simulink model "AirCooledDataCenterTemperatureProfile"  (R2025b)
settings: Solver=daessc  StartTime=0.0  StopTime=24*3600  MaxStep=1  RelTol=1e-3  AbsTol=1e-3
PreLoadFcn:
  | if ~exist("airCooledDataCenter")
  |     setModelParam;
  | end
undefined symbols (not defined in the file or in its folder): airCooledDataCenter, DiscIntNeverNeededParam, value
libraries: fl_lib x166, nesl_utility x25, datacenter_lib x24, simulink_extras x9
(part 1 of 4)
settings Model: Creator=vikrants  LastModifiedBy=vikrants
settings SolverCC: AutoScaleAbsTol=off  MaxConsecutiveMinStep=3  AlgebraicLoopSolver=TrustRegion  MaxZcPerStep=1.0
settings DataIOCC: SaveOutput=off  DSMLogging=off  SaveTime=off  ReturnWorkspaceOutputs=off  SignalLoggingName=logsout_AirCooledDataCenterTprofile
settings DebuggingCC: UnconnectedInputMsg=warning  UnconnectedOutputMsg=warning  UnconnectedLineMsg=warning  SymbolicDimsDataTypeCodeGenerationDiagnostic=none
settings ModelReferenceCC: EnableRefExpFcnMdlSchedulingChecks=on
settings SFSimCC: CustomCodeUndefinedFunction=UseInterfaceOnly
settings RTWCC: GPUComputeCapability=3.5  DLArmComputeVersion=19.05
settings SimscapeCC: SimscapeLogSimulationStatistics=on  SimscapeLogDataHistory=10000.0

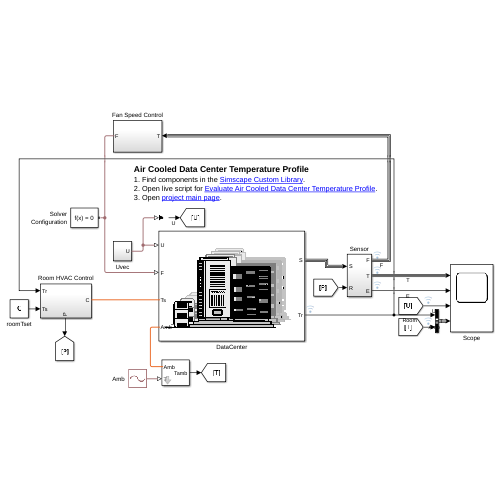
[thumbnail: Simulink's stored preview of the top-level diagram]
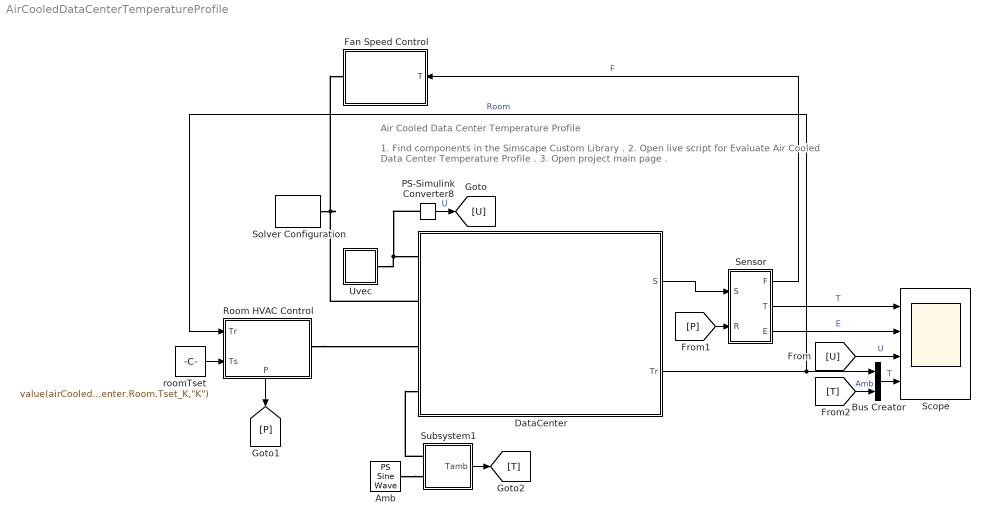
== system AirCooledDataCenterTemperatureProfile ==
  note: Air Cooled Data Center Temperature Profile
  note: 1. Find components in the Simscape Custom Library .
      | 2. Open live script for Evaluate Air Cooled Data Center Temperature Profile .
      | 3. Open project main page .
  Amb : fl_lib/Physical Signals/Sources/PS Sine Wave  amplitude=1 K  bias="value(airCooledDataCenter.HeatTransfer.AmbientT,\"K\") K"  frequency_spec=foundation.enum.frequencySpec.frequencySI  frequency_SI=1/3600 Hz  frequency_angular=1 rad/s  phase=0 rad
      settings: InternalSimscapePortConfiguration="{\"Bottom\":[],\"Left\":[],\"Right\":[{\"id\":\"O\",\"label\":\"\",\"type\":\"output\"}],\"Top\":[]}"
  Bus Creator : BusCreator  Inputs=2
  DataCenter : Subsystem
      mask Display: image('datacenterLibIcon.png');
  Fan Speed Control : Subsystem
      settings: PortSchema="{\"entries\":[{\"content\":{\"sides\":[{\"content\":{\"connectorIds\":[\"LConn1\"]},\"type\":\"ConnectorPlacement.EquallySpacedRectSide\",\"uuid\":\"25bb085d-e973-4ed5-b016-3236384605d7\"},{\"content\":{\"connectorIds\":[\"In1\"],\"side\":\"RIGHT\"},\"type\":\"ConnectorPlacement.EquallySpacedRectSide\",\"uuid\":\"9c70bb1c-0b86-445b-9231-deb3b11a43cd\"},{\"content\":{\"side\":\"TOP\"},\"type\":\"ConnectorPlacement.EquallySpacedRectSide\",\"uuid\":\"a44df08c-50be-4908-a6d5-8f6a23919272\"}]},\"type\":\"ConnectorPlacement.EquallySpacedConnector\",\"uuid\":\"adee43dd-4b72-4470-a633-4adaea9baf7d\"}],\"packageUris\":[\"http://schema.mathworks.com/mf0/Connector/R2020b\"],\"version\":\"1.0\"}"
  PS-Simulink Converter8 : nesl_utility/PS-Simulink Converter  PhysicalDomain=network_engine_domain  SubClassName=ps_output  LeftPortType=input  RightPortType=output  PseudoPeriodic=off  Frequencies=[]  VectorFormat=inherit  Unit=inherit  AffineConversion=off
  Room HVAC Control : Subsystem
      settings: PortSchema="{\"entries\":[{\"content\":{\"sides\":[{\"content\":{\"connectorIds\":[\"In1\",\"In2\"]},\"type\":\"ConnectorPlacement.EquallySpacedRectSide\",\"uuid\":\"3724864a-83d6-4228-951d-7164f41f00c6\"},{\"content\":{\"connectorIds\":[\"RConn1\"],\"side\":\"RIGHT\"},\"type\":\"ConnectorPlacement.EquallySpacedRectSide\",\"uuid\":\"0a482fb7-33c2-448f-90c4-95efee70f83f\"},{\"content\":{\"side\":\"TOP\"},\"type\":\"ConnectorPlacement.EquallySpacedRectSide\",\"uuid\":\"deb1033d-adc7-41d0-9927-16876749a2b1\"},{\"content\":{\"connectorIds\":[\"Out1\"],\"side\":\"BOTTOM\"},\"type\":\"ConnectorPlacement.EquallySpacedRectSide\",\"uuid\":\"12511515-206f-4008-b3c0-49360f108e7c\"}]},\"type\":\"ConnectorPlacement.EquallySpacedConnector\",\"uuid\":\"be3e27ef-0111-44f1-89d2-5affe53329b4\"}],\"packageUris\":[\"http://schema.mathworks.com/mf0/Connector/R2020b\"],\"version\":\"1.0\"}"
  Scope : Scope  NumInputPorts=4
      settings: ActiveDisplayYMinimum=-123.69235993685102  ActiveDisplayYMaximum=1124.8547066596502
  Sensor : Subsystem
  Solver Configuration : nesl_utility/Solver Configuration  PhysicalDomain=network_engine_domain  SubClassName=solver  LeftPortType=input  RightPortType=generic  Tones=[]  Harmonics=[]  SimulateNoise=off  Profile=off  UseLocalSampling=off  EnableSwitchedLinearOptims=on  FrequencyDomain=off  UseCCode=off  RelTol=0.001  AbsTol=1e-06  MinStep=1e-09  ToWorkspace=off  RevertToSquareIcSolve=off  NumHomotopyIterations=100  PhasorMode=off  PhasorModeNumHarmonics=1  ConsistencySolver=NEWTON_XTOL_AFTER_FTOL  IndexReductionMethod=DerivativeReplacement  DoDC=off  ResidualTolerance=1e-09  ConsistencyTolSource=GLOBAL  ConsistencyAbsTol=0.001  ConsistencyRelTol=0.001  ConsistencyTolFactor=0.001  UseLocalSolver=off  LocalSolverChoice=NE_BACKWARD_EULER_ADVANCER  ResolveIndetEquations=on  FunctionEvalNumThread=1  LocalSolverSampleTime=0.001  DoFixedCost=off  MaxNonlinIter=3  MaxModeIter=2  ComputeImpulses=off  ImpulseIterations=2  LinearAlgebra=auto  LinearAlgebraNumThread=0  EquationFormulation=NE_TIME_EF  DelaysMemoryBudget=1024  AutomaticFiltering=on  FilteringTimeConstant=0.001  PartitionStorageMethod=AS_NEEDED  PartitionMemoryBudget=1024  PartitionMethod=ROBUST  MultibodyUseLocalSolver=off  MultibodyLocalSolverChoice=ODE1  MultibodyLocalSolverSampleTime=0.001
  Subsystem1 : Subsystem  mask{thermalR=0.01}
      mask prompts: thermalR "Thermal resistance (K/W)"
  Uvec : Subsystem
  roomTset : Constant  Value="value(airCooledDataCenter.Room.Tset_K,\"K\")"
  wires:
  DataCenter/1(S) -> Sensor/1(S)
  Sensor/2(T) -> Scope/1  "T"
  Sensor/3(E) -> Scope/2  "E"
  Sensor/1(F) -> Fan Speed Control/1(T)  "F"
  PS-Simulink Converter8/1 -> [U]  "U"
  [U] -> Scope/3  "U"
  DataCenter/2(Tr) -> Bus Creator/1, Room HVAC Control/1(Tr)  "Room"
  Subsystem1/1(Tamb) -> [T]
  [T] -> Bus Creator/2  "Amb"
  Bus Creator/1 -> Scope/4  "T"
  roomTset/1 -> Room HVAC Control/2(Ts)
  Room HVAC Control/1(P) -> [P]
  [P] -> Sensor/2(R)
  connections:
  Uvec/RConn1 -- PS-Simulink Converter8/LConn1 -- DataCenter/LConn1
  DataCenter/LConn2 -- Fan Speed Control/LConn1 -- Solver Configuration/RConn1
  Subsystem1/LConn1 -- DataCenter/LConn4
  Amb/RConn1 -- Subsystem1/LConn2
  Room HVAC Control/RConn1 -- DataCenter/LConn3

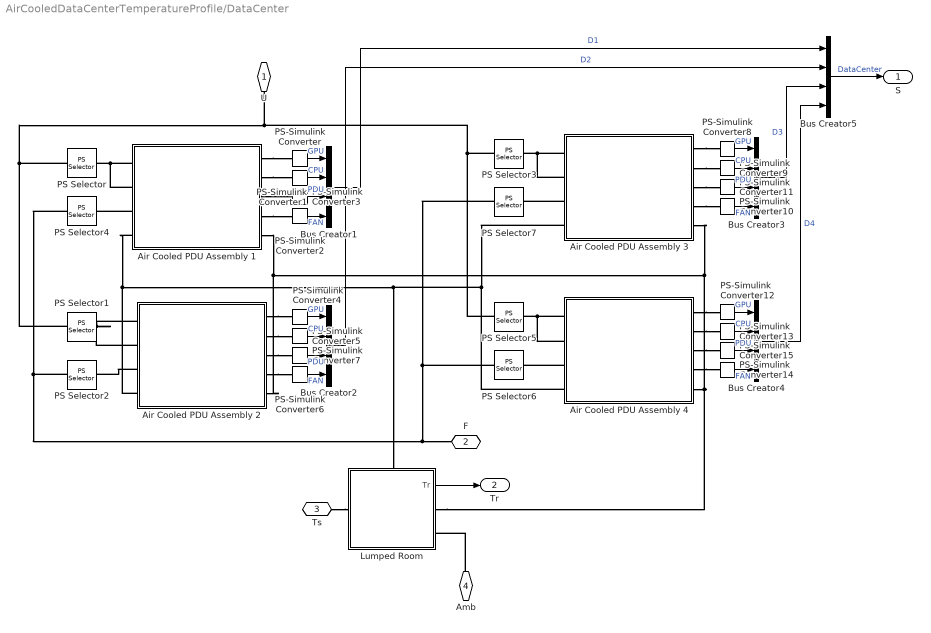
== system AirCooledDataCenterTemperatureProfile/DataCenter ==
  Air Cooled PDU Assembly 1 : Subsystem  mask{nAssembly=1, nRacks=4, nTrays=6, nFans=36, flowVec=[500:250:1500]*0.000472, prDropVec=[7000:250:8000], fanEffVec=[0.88, 0.89, 0.90, 0.895, 0.89], trayMass=8, trayCp=8000, trayThermalR=1e-3, nGPU=4, gpuTDPperDie=1200, gpuIdlePower=300, gpuHBMpower=80, gpuExponent=1.4, gpuHBMutil=0.7, gpuLeakage=1.5, gpuNominalDieT=350, gpuDieThermalC=50, gpuHeatSinkR=1e-3, gpuSurfArea=0.01, gpuAmbientR=1e-3, nCPU=2, cpuTDPperSocket=350, cpuIdlePower=80, cpuExponent=1.1, cpuLeakage=1.5, cpuNominalDieT=350, cpuDieThermalC=50, cpuHeatSinkR=1e-3, cpuSurfArea=0.01, cpuAmbientR=1e-3, initialT=value(airCooledDataCenter.HeatTransfer.InitialT,"K"), htc=value(airCooledDataCenter.HeatTransfer.HTC,"W/(K*m^2)")}
      mask prompts: nAssembly "Number of PDU + Fan assemblies (-)"; nRacks "Number of racks per PDU (-)"; nTrays "Number of IT trays per rack (-)"; nFans "Number of fans per assembly (-)"; flowVec "Fan flow rate vector (m^3/s)"; prDropVec "Fan pressure drop vector (Pa)"; fanEffVec "Fan efficiency vector, 0-1 (-)"; trayMass "Tray mass (kg)"; trayCp "Tray specific heat capacity (J/kg*K)"; trayThermalR "Tray to external thermal resistance (K/W)"; nGPU "Number of GPU per tray (-)"; gpuTDPperDie "GPU TDP per die (W)"; gpuIdlePower "GPU idle power (W)"; gpuHBMpower "HBM power per GPU (W)"; gpuExponent "GPU power utilization exponent (-)"; gpuHBMutil "HBM utilization as fraction of compute utilization (-)"; gpuLeakage "Leakage increase per K above nominal temperature (W/K)"; gpuNominalDieT "Nominal die temperature at TDP (K)"; gpuDieThermalC "GPU die thermal capacitance (J/K)"; gpuHeatSinkR "GPU die-heat-sink thermal resistance (K/W)"; gpuSurfArea "Surface area per die for ambient heat transfer (m^2)"; gpuAmbientR "GPU die-ambient thermal resistance (K/W)"; nCPU "Number of CPU per tray (-)"; cpuTDPperSocket "CPU TDP per socket (W)"; cpuIdlePower "CPU idle power per socket (W)"; cpuExponent "CPU power utilization exponent (-)"; cpuLeakage "Leakage increase per K above nominal temperature (W/K)"; cpuNominalDieT "Nominal die temperature at TDP (K)"; cpuDieThermalC "CPU die thermal capacitance (J/K)"; cpuHeatSinkR "CPU die-heat-sink thermal resistance (K/W)"; cpuSurfArea "Surface area per die for ambient heat transfer (m^2)"; cpuAmbientR "CPU die-ambient thermal resistance (K/W)"; initialT "Initial temperature (K)"; htc "Heat transfer coefficient to ambient (W/m^2.K)"
      settings: CopyFcn=set_param(gcbh,'LinkStatus','none');
      mask Help: web("DocumentationAirCooledPDUAssembly.html")
      mask DialogControl Container10 Prompt: PDU Racks
      mask DialogControl getRatingButton Prompt: Get Rating
      mask DialogControl Container11 Prompt: Fans
      mask DialogControl Container9 Prompt: IT Tray
      mask DialogControl Container6 Prompt: GPU
      mask DialogControl Container7 Prompt: CPU
      mask DialogControl Container8 Prompt: Initial Conditions
      mask Display: image('icon_AssemblyAirCooled.png');
  Air Cooled PDU Assembly 2 : Subsystem  mask{nAssembly=1, nRacks=4, nTrays=6, nFans=36, flowVec=[500:250:1500]*0.000472, prDropVec=[7000:250:8000], fanEffVec=[0.88, 0.89, 0.90, 0.895, 0.89], trayMass=8, trayCp=8000, trayThermalR=1e-3, nGPU=4, gpuTDPperDie=1200, gpuIdlePower=300, gpuHBMpower=80, gpuExponent=1.4, gpuHBMutil=0.7, gpuLeakage=1.5, gpuNominalDieT=350, gpuDieThermalC=50, gpuHeatSinkR=1e-3, gpuSurfArea=0.01, gpuAmbientR=1e-3, nCPU=2, cpuTDPperSocket=350, cpuIdlePower=80, cpuExponent=1.1, cpuLeakage=1.5, cpuNominalDieT=350, cpuDieThermalC=50, cpuHeatSinkR=1e-3, cpuSurfArea=0.01, cpuAmbientR=1e-3, initialT=value(airCooledDataCenter.HeatTransfer.InitialT,"K"), htc=value(airCooledDataCenter.HeatTransfer.HTC,"W/(K*m^2)")}
      mask prompts: nAssembly "Number of PDU + Fan assemblies (-)"; nRacks "Number of racks per PDU (-)"; nTrays "Number of IT trays per rack (-)"; nFans "Number of fans per assembly (-)"; flowVec "Fan flow rate vector (m^3/s)"; prDropVec "Fan pressure drop vector (Pa)"; fanEffVec "Fan efficiency vector, 0-1 (-)"; trayMass "Tray mass (kg)"; trayCp "Tray specific heat capacity (J/kg*K)"; trayThermalR "Tray to external thermal resistance (K/W)"; nGPU "Number of GPU per tray (-)"; gpuTDPperDie "GPU TDP per die (W)"; gpuIdlePower "GPU idle power (W)"; gpuHBMpower "HBM power per GPU (W)"; gpuExponent "GPU power utilization exponent (-)"; gpuHBMutil "HBM utilization as fraction of compute utilization (-)"; gpuLeakage "Leakage increase per K above nominal temperature (W/K)"; gpuNominalDieT "Nominal die temperature at TDP (K)"; gpuDieThermalC "GPU die thermal capacitance (J/K)"; gpuHeatSinkR "GPU die-heat-sink thermal resistance (K/W)"; gpuSurfArea "Surface area per die for ambient heat transfer (m^2)"; gpuAmbientR "GPU die-ambient thermal resistance (K/W)"; nCPU "Number of CPU per tray (-)"; cpuTDPperSocket "CPU TDP per socket (W)"; cpuIdlePower "CPU idle power per socket (W)"; cpuExponent "CPU power utilization exponent (-)"; cpuLeakage "Leakage increase per K above nominal temperature (W/K)"; cpuNominalDieT "Nominal die temperature at TDP (K)"; cpuDieThermalC "CPU die thermal capacitance (J/K)"; cpuHeatSinkR "CPU die-heat-sink thermal resistance (K/W)"; cpuSurfArea "Surface area per die for ambient heat transfer (m^2)"; cpuAmbientR "CPU die-ambient thermal resistance (K/W)"; initialT "Initial temperature (K)"; htc "Heat transfer coefficient to ambient (W/m^2.K)"
      settings: CopyFcn=set_param(gcbh,'LinkStatus','none');
      mask Help: web("DocumentationAirCooledPDUAssembly.html")
      mask DialogControl Container10 Prompt: PDU Racks
      mask DialogControl getRatingButton Prompt: Get Rating
      mask DialogControl Container11 Prompt: Fans
      mask DialogControl Container9 Prompt: IT Tray
      mask DialogControl Container6 Prompt: GPU
      mask DialogControl Container7 Prompt: CPU
      mask DialogControl Container8 Prompt: Initial Conditions
      mask Display: image('icon_AssemblyAirCooled.png');
  Air Cooled PDU Assembly 3 : Subsystem  mask{nAssembly=1, nRacks=4, nTrays=6, nFans=36, flowVec=[500:250:1500]*0.000472, prDropVec=[7000:250:8000], fanEffVec=[0.88, 0.89, 0.90, 0.895, 0.89], trayMass=8, trayCp=8000, trayThermalR=1e-3, nGPU=4, gpuTDPperDie=1200, gpuIdlePower=300, gpuHBMpower=80, gpuExponent=1.4, gpuHBMutil=0.7, gpuLeakage=1.5, gpuNominalDieT=350, gpuDieThermalC=50, gpuHeatSinkR=1e-3, gpuSurfArea=0.01, gpuAmbientR=1e-3, nCPU=2, cpuTDPperSocket=350, cpuIdlePower=80, cpuExponent=1.1, cpuLeakage=1.5, cpuNominalDieT=350, cpuDieThermalC=50, cpuHeatSinkR=1e-3, cpuSurfArea=0.01, cpuAmbientR=1e-3, initialT=value(airCooledDataCenter.HeatTransfer.InitialT,"K"), htc=value(airCooledDataCenter.HeatTransfer.HTC,"W/(K*m^2)")}
      mask prompts: nAssembly "Number of PDU + Fan assemblies (-)"; nRacks "Number of racks per PDU (-)"; nTrays "Number of IT trays per rack (-)"; nFans "Number of fans per assembly (-)"; flowVec "Fan flow rate vector (m^3/s)"; prDropVec "Fan pressure drop vector (Pa)"; fanEffVec "Fan efficiency vector, 0-1 (-)"; trayMass "Tray mass (kg)"; trayCp "Tray specific heat capacity (J/kg*K)"; trayThermalR "Tray to external thermal resistance (K/W)"; nGPU "Number of GPU per tray (-)"; gpuTDPperDie "GPU TDP per die (W)"; gpuIdlePower "GPU idle power (W)"; gpuHBMpower "HBM power per GPU (W)"; gpuExponent "GPU power utilization exponent (-)"; gpuHBMutil "HBM utilization as fraction of compute utilization (-)"; gpuLeakage "Leakage increase per K above nominal temperature (W/K)"; gpuNominalDieT "Nominal die temperature at TDP (K)"; gpuDieThermalC "GPU die thermal capacitance (J/K)"; gpuHeatSinkR "GPU die-heat-sink thermal resistance (K/W)"; gpuSurfArea "Surface area per die for ambient heat transfer (m^2)"; gpuAmbientR "GPU die-ambient thermal resistance (K/W)"; nCPU "Number of CPU per tray (-)"; cpuTDPperSocket "CPU TDP per socket (W)"; cpuIdlePower "CPU idle power per socket (W)"; cpuExponent "CPU power utilization exponent (-)"; cpuLeakage "Leakage increase per K above nominal temperature (W/K)"; cpuNominalDieT "Nominal die temperature at TDP (K)"; cpuDieThermalC "CPU die thermal capacitance (J/K)"; cpuHeatSinkR "CPU die-heat-sink thermal resistance (K/W)"; cpuSurfArea "Surface area per die for ambient heat transfer (m^2)"; cpuAmbientR "CPU die-ambient thermal resistance (K/W)"; initialT "Initial temperature (K)"; htc "Heat transfer coefficient to ambient (W/m^2.K)"
      settings: CopyFcn=set_param(gcbh,'LinkStatus','none');
      mask Help: web("DocumentationAirCooledPDUAssembly.html")
      mask DialogControl Container10 Prompt: PDU Racks
      mask DialogControl getRatingButton Prompt: Get Rating
      mask DialogControl Container11 Prompt: Fans
      mask DialogControl Container9 Prompt: IT Tray
      mask DialogControl Container6 Prompt: GPU
      mask DialogControl Container7 Prompt: CPU
      mask DialogControl Container8 Prompt: Initial Conditions
      mask Display: image('icon_AssemblyAirCooled.png');
  Air Cooled PDU Assembly 4 : Subsystem  mask{nAssembly=1, nRacks=4, nTrays=6, nFans=36, flowVec=[500:250:1500]*0.000472, prDropVec=[7000:250:8000], fanEffVec=[0.88, 0.89, 0.90, 0.895, 0.89], trayMass=8, trayCp=8000, trayThermalR=1e-3, nGPU=4, gpuTDPperDie=1200, gpuIdlePower=300, gpuHBMpower=80, gpuExponent=1.4, gpuHBMutil=0.7, gpuLeakage=1.5, gpuNominalDieT=350, gpuDieThermalC=50, gpuHeatSinkR=1e-3, gpuSurfArea=0.01, gpuAmbientR=1e-3, nCPU=2, cpuTDPperSocket=350, cpuIdlePower=80, cpuExponent=1.1, cpuLeakage=1.5, cpuNominalDieT=350, cpuDieThermalC=50, cpuHeatSinkR=1e-3, cpuSurfArea=0.01, cpuAmbientR=1e-3, initialT=value(airCooledDataCenter.HeatTransfer.InitialT,"K"), htc=value(airCooledDataCenter.HeatTransfer.HTC,"W/(K*m^2)")}
      mask prompts: nAssembly "Number of PDU + Fan assemblies (-)"; nRacks "Number of racks per PDU (-)"; nTrays "Number of IT trays per rack (-)"; nFans "Number of fans per assembly (-)"; flowVec "Fan flow rate vector (m^3/s)"; prDropVec "Fan pressure drop vector (Pa)"; fanEffVec "Fan efficiency vector, 0-1 (-)"; trayMass "Tray mass (kg)"; trayCp "Tray specific heat capacity (J/kg*K)"; trayThermalR "Tray to external thermal resistance (K/W)"; nGPU "Number of GPU per tray (-)"; gpuTDPperDie "GPU TDP per die (W)"; gpuIdlePower "GPU idle power (W)"; gpuHBMpower "HBM power per GPU (W)"; gpuExponent "GPU power utilization exponent (-)"; gpuHBMutil "HBM utilization as fraction of compute utilization (-)"; gpuLeakage "Leakage increase per K above nominal temperature (W/K)"; gpuNominalDieT "Nominal die temperature at TDP (K)"; gpuDieThermalC "GPU die thermal capacitance (J/K)"; gpuHeatSinkR "GPU die-heat-sink thermal resistance (K/W)"; gpuSurfArea "Surface area per die for ambient heat transfer (m^2)"; gpuAmbientR "GPU die-ambient thermal resistance (K/W)"; nCPU "Number of CPU per tray (-)"; cpuTDPperSocket "CPU TDP per socket (W)"; cpuIdlePower "CPU idle power per socket (W)"; cpuExponent "CPU power utilization exponent (-)"; cpuLeakage "Leakage increase per K above nominal temperature (W/K)"; cpuNominalDieT "Nominal die temperature at TDP (K)"; cpuDieThermalC "CPU die thermal capacitance (J/K)"; cpuHeatSinkR "CPU die-heat-sink thermal resistance (K/W)"; cpuSurfArea "Surface area per die for ambient heat transfer (m^2)"; cpuAmbientR "CPU die-ambient thermal resistance (K/W)"; initialT "Initial temperature (K)"; htc "Heat transfer coefficient to ambient (W/m^2.K)"
      settings: CopyFcn=set_param(gcbh,'LinkStatus','none');
      mask Help: web("DocumentationAirCooledPDUAssembly.html")
      mask DialogControl Container10 Prompt: PDU Racks
      mask DialogControl getRatingButton Prompt: Get Rating
      mask DialogControl Container11 Prompt: Fans
      mask DialogControl Container9 Prompt: IT Tray
      mask DialogControl Container6 Prompt: GPU
      mask DialogControl Container7 Prompt: CPU
      mask DialogControl Container8 Prompt: Initial Conditions
      mask Display: image('icon_AssemblyAirCooled.png');
  Bus Creator{1..5} (5 alike) : BusCreator  Inputs=4
  Lumped Room : Subsystem  mask{len=value(airCooledDataCenter.Room.Length,"m"), wid=value(airCooledDataCenter.Room.Width,"m"), hgt=value(airCooledDataCenter.Room.Height,"m"), pc=airCooledDataCenter.Room.RoomAssetVolPercent, htc=value(airCooledDataCenter.HeatTransfer.HTC,"W/(K*m^2)"), iniT=value(airCooledDataCenter.HeatTransfer.InitialT,"K")}
      mask prompts: len "Length (m)"; wid "Width (m)"; hgt "Height (m)"; pc "Percent room volume occupied by data centers (%)"; htc "Heat transfer coefficient (W/(m^2.K))"; iniT "Initial temperature (K)"
      settings: PortSchema="{\"entries\":[{\"content\":{\"sides\":[{\"content\":{\"connectorIds\":[\"LConn1\"]},\"type\":\"ConnectorPlacement.EquallySpacedRectSide\",\"uuid\":\"f266d7ff-208e-47ff-9cdb-67d745596a07\"},{\"content\":{\"connectorIds\":[\"Out1\",\"RConn1\",\"RConn2\"],\"side\":\"RIGHT\"},\"type\":\"ConnectorPlacement.EquallySpacedRectSide\",\"uuid\":\"8ecfba95-8c7d-4766-9064-e345a76ffd27\"},{\"content\":{\"connectorIds\":[\"LConn2\"],\"side\":\"TOP\"},\"type\":\"ConnectorPlacement.EquallySpacedRectSide\",\"uuid\":\"d31bb3e3-0ab2-4c01-ad1d-6bcb628ec073\"}]},\"type\":\"ConnectorPlacement.EquallySpacedConnector\",\"uuid\":\"b60a5775-7ee8-4e86-b260-6d90d09432cb\"}],\"packageUris\":[\"http://schema.mathworks.com/mf0/Connector/R2020b\"],\"version\":\"1.0\"}"
      mask DialogControl Container2 Prompt: Room Dimensions
      mask DialogControl Container3 Prompt: Heat Transfer
  PS Selector : fl_lib/Physical Signals/Nonlinear Operators/PS Selector  ix=1
      settings: InternalSimscapePortConfiguration="{\"Bottom\":[],\"Left\":[{\"id\":\"I\",\"label\":\"\",\"type\":\"input\"}],\"Right\":[{\"id\":\"O\",\"label\":\"\",\"type\":\"output\"}],\"Top\":[]}"
  PS Selector1 : fl_lib/Physical Signals/Nonlinear Operators/PS Selector  ix=2
      settings: InternalSimscapePortConfiguration="{\"Bottom\":[],\"Left\":[{\"id\":\"I\",\"label\":\"\",\"type\":\"input\"}],\"Right\":[{\"id\":\"O\",\"label\":\"\",\"type\":\"output\"}],\"Top\":[]}"
  PS Selector2 : fl_lib/Physical Signals/Nonlinear Operators/PS Selector  ix=2
      settings: InternalSimscapePortConfiguration="{\"Bottom\":[],\"Left\":[{\"id\":\"I\",\"label\":\"\",\"type\":\"input\"}],\"Right\":[{\"id\":\"O\",\"label\":\"\",\"type\":\"output\"}],\"Top\":[]}"
  PS Selector3 : fl_lib/Physical Signals/Nonlinear Operators/PS Selector  ix=3
      settings: InternalSimscapePortConfiguration="{\"Bottom\":[],\"Left\":[{\"id\":\"I\",\"label\":\"\",\"type\":\"input\"}],\"Right\":[{\"id\":\"O\",\"label\":\"\",\"type\":\"output\"}],\"Top\":[]}"
  PS Selector4 : fl_lib/Physical Signals/Nonlinear Operators/PS Selector  ix=1
      settings: InternalSimscapePortConfiguration="{\"Bottom\":[],\"Left\":[{\"id\":\"I\",\"label\":\"\",\"type\":\"input\"}],\"Right\":[{\"id\":\"O\",\"label\":\"\",\"type\":\"output\"}],\"Top\":[]}"
  PS Selector5 : fl_lib/Physical Signals/Nonlinear Operators/PS Selector  ix=4
      settings: InternalSimscapePortConfiguration="{\"Bottom\":[],\"Left\":[{\"id\":\"I\",\"label\":\"\",\"type\":\"input\"}],\"Right\":[{\"id\":\"O\",\"label\":\"\",\"type\":\"output\"}],\"Top\":[]}"
  PS Selector6 : fl_lib/Physical Signals/Nonlinear Operators/PS Selector  ix=4
      settings: InternalSimscapePortConfiguration="{\"Bottom\":[],\"Left\":[{\"id\":\"I\",\"label\":\"\",\"type\":\"input\"}],\"Right\":[{\"id\":\"O\",\"label\":\"\",\"type\":\"output\"}],\"Top\":[]}"
  PS Selector7 : fl_lib/Physical Signals/Nonlinear Operators/PS Selector  ix=3
      settings: InternalSimscapePortConfiguration="{\"Bottom\":[],\"Left\":[{\"id\":\"I\",\"label\":\"\",\"type\":\"input\"}],\"Right\":[{\"id\":\"O\",\"label\":\"\",\"type\":\"output\"}],\"Top\":[]}"
  PS-Simulink Converter{,1..15} (16 alike) : nesl_utility/PS-Simulink Converter  PhysicalDomain=network_engine_domain  SubClassName=ps_output  LeftPortType=input  RightPortType=output  PseudoPeriodic=off  Frequencies=[]  VectorFormat=inherit  Unit=inherit  AffineConversion=off
  U : PMIOPort  Side=Left
  F : PMIOPort  Port=2  Side=Left
  Ts : PMIOPort  Port=3  Side=Left
  Amb : PMIOPort  Port=4  Side=Left
  S : Outport
  Tr : Outport  Port=2
  wires:
  PS-Simulink Converter14/1 -> Bus Creator4/4  "FAN"
  PS-Simulink Converter4/1 -> Bus Creator2/1  "GPU"
  PS-Simulink Converter12/1 -> Bus Creator4/1  "GPU"
  PS-Simulink Converter6/1 -> Bus Creator2/4  "FAN"
  PS-Simulink Converter7/1 -> Bus Creator2/3  "PDU"
  PS-Simulink Converter5/1 -> Bus Creator2/2  "CPU"
  PS-Simulink Converter1/1 -> Bus Creator1/2  "CPU"
  PS-Simulink Converter9/1 -> Bus Creator3/2  "CPU"
  PS-Simulink Converter/1 -> Bus Creator1/1  "GPU"
  PS-Simulink Converter8/1 -> Bus Creator3/1  "GPU"
  PS-Simulink Converter15/1 -> Bus Creator4/3  "PDU"
  PS-Simulink Converter11/1 -> Bus Creator3/3  "PDU"
  PS-Simulink Converter2/1 -> Bus Creator1/4  "FAN"
  PS-Simulink Converter3/1 -> Bus Creator1/3  "PDU"
  PS-Simulink Converter10/1 -> Bus Creator3/4  "FAN"
  PS-Simulink Converter13/1 -> Bus Creator4/2  "CPU"
  Bus Creator3/1 -> Bus Creator5/3  "D3"
  Bus Creator4/1 -> Bus Creator5/4  "D4"
  Bus Creator2/1 -> Bus Creator5/2  "D2"
  Bus Creator1/1 -> Bus Creator5/1  "D1"
  Bus Creator5/1 -> S/1  "DataCenter"
  Lumped Room/1(Tr) -> Tr/1
  connections:
  Air Cooled PDU Assembly 3/RConn1 -- PS-Simulink Converter8/LConn1
  Air Cooled PDU Assembly 4/RConn4 -- PS-Simulink Converter14/LConn1
  Air Cooled PDU Assembly 1/LConn3 -- PS Selector4/RConn1
  Air Cooled PDU Assembly 1/RConn3 -- PS-Simulink Converter3/LConn1
  PS Selector/RConn1 -- Air Cooled PDU Assembly 1/LConn1 -- Air Cooled PDU Assembly 1/LConn2
  Air Cooled PDU Assembly 3/LConn3 -- PS Selector7/RConn1
  PS Selector1/RConn1 -- Air Cooled PDU Assembly 2/LConn2 -- Air Cooled PDU Assembly 2/LConn1
  Air Cooled PDU Assembly 3/RConn3 -- PS-Simulink Converter11/LConn1
  Air Cooled PDU Assembly 3/RConn2 -- PS-Simulink Converter9/LConn1
  Air Cooled PDU Assembly 2/RConn1 -- PS-Simulink Converter4/LConn1
  Air Cooled PDU Assembly 3/RConn4 -- PS-Simulink Converter10/LConn1
  PS Selector/LConn1 -- PS Selector1/LConn1 -- PS Selector5/LConn1 -- PS Selector3/LConn1 -- U/RConn1
  PS Selector7/LConn1 -- PS Selector6/LConn1 -- PS Selector2/LConn1 -- PS Selector4/LConn1 -- F/RConn1
  Air Cooled PDU Assembly 1/RConn4 -- PS-Simulink Converter2/LConn1
  Air Cooled PDU Assembly 2/RConn3 -- PS-Simulink Converter7/LConn1
  PS Selector3/RConn1 -- Air Cooled PDU Assembly 3/LConn1 -- Air Cooled PDU Assembly 3/LConn2
  PS Selector5/RConn1 -- Air Cooled PDU Assembly 4/LConn1 -- Air Cooled PDU Assembly 4/LConn2
  Air Cooled PDU Assembly 1/RConn2 -- PS-Simulink Converter1/LConn1
  Air Cooled PDU Assembly 4/LConn3 -- PS Selector6/RConn1
  Air Cooled PDU Assembly 2/RConn2 -- PS-Simulink Converter5/LConn1
  Air Cooled PDU Assembly 1/RConn1 -- PS-Simulink Converter/LConn1
  Air Cooled PDU Assembly 4/RConn2 -- PS-Simulink Converter13/LConn1
  Air Cooled PDU Assembly 4/RConn1 -- PS-Simulink Converter12/LConn1
  Air Cooled PDU Assembly 4/RConn3 -- PS-Simulink Converter15/LConn1
  Air Cooled PDU Assembly 2/RConn4 -- PS-Simulink Converter6/LConn1
  Air Cooled PDU Assembly 2/LConn3 -- PS Selector2/RConn1
  Air Cooled PDU Assembly 3/LConn4 -- Air Cooled PDU Assembly 4/LConn4 -- Lumped Room/LConn2 -- Air Cooled PDU Assembly 2/LConn4 -- Air Cooled PDU Assembly 1/LConn4
  Air Cooled PDU Assembly 2/RConn5 -- Air Cooled PDU Assembly 1/RConn5 -- Air Cooled PDU Assembly 3/RConn5 -- Air Cooled PDU Assembly 4/RConn5 -- Lumped Room/RConn1
  Ts/RConn1 -- Lumped Room/LConn1
  Amb/RConn1 -- Lumped Room/RConn2

== system AirCooledDataCenterTemperatureProfile/Fan Speed Control ==
  T : Inport
  Subsystem4 : Subsystem
  Subsystem5 : Subsystem  mask{measDelay=1, upperT=value(airCooledDataCenter.Fan.UpperT,"K"), lowerT=value(airCooledDataCenter.Fan.LowerT,"K")}
      mask prompts: measDelay "Measurement delay (s)"; upperT "Upper limit for temperature control (K)"; lowerT "Lower limit for temperature control (K)"
      settings: PortSchema="{\"entries\":[{\"content\":{\"sides\":[{\"content\":{\"connectorIds\":[\"LConn1\",\"LConn2\",\"LConn3\",\"LConn4\"]},\"type\":\"ConnectorPlacement.EquallySpacedRectSide\",\"uuid\":\"b9d7e346-d2bb-4aef-805d-3c70223bcabc\"},{\"content\":{\"connectorIds\":[\"In1\"],\"side\":\"RIGHT\"},\"type\":\"ConnectorPlacement.EquallySpacedRectSide\",\"uuid\":\"897d6b10-2a91-4282-b9ce-e7b5d2f48be3\"},{\"content\":{\"side\":\"TOP\"},\"type\":\"ConnectorPlacement.EquallySpacedRectSide\",\"uuid\":\"85a41cbf-50a8-4390-990a-3b28562dd1ba\"}]},\"type\":\"ConnectorPlacement.EquallySpacedConnector\",\"uuid\":\"8275b9c6-e30f-4962-88f8-e8477ac76c6b\"}],\"packageUris\":[\"http://schema.mathworks.com/mf0/Connector/R2020b\"],\"version\":\"1.0\"}"
  F : PMIOPort  Side=Left
  wires:
  T/1 -> Subsystem5/1(T)
  connections:
  Subsystem4/RConn1 -- F/RConn1
  Subsystem4/LConn4 -- Subsystem5/LConn1
  Subsystem5/LConn2 -- Subsystem4/LConn3
  Subsystem5/LConn3 -- Subsystem4/LConn2
  Subsystem5/LConn4 -- Subsystem4/LConn1

== system AirCooledDataCenterTemperatureProfile/Room HVAC Control ==
  Tr : Inport
  Ts : Inport  Port=2
  Room HVAC : Subsystem  mask{effHeatExchanger=airCooledDataCenter.Room.HVAC.EffHeatExchanger, tLag=1, roomLen=value(airCooledDataCenter.Room.Length,"m"), roomWid=value(airCooledDataCenter.Room.Width,"m"), roomHt=value(airCooledDataCenter.Room.Height,"m"), fracRoomVolDC=airCooledDataCenter.Room.RoomAssetVolPercent/100}
      mask prompts: effHeatExchanger "Efficiency (%)"; tLag "Measurement delay (s)"; roomLen "Length (m)"; roomWid "Width (m)"; roomHt "Height (m)"; fracRoomVolDC "Fraction of room volume occupied by data center (-)"
      mask DialogControl Container3 Prompt: Heat Exchanger
      mask DialogControl Container2 Prompt: Room Details
  Subsystem : Subsystem
      settings: PortSchema="{\"entries\":[{\"content\":{\"sides\":[{\"content\":{\"connectorIds\":[\"In1\"]},\"type\":\"ConnectorPlacement.EquallySpacedRectSide\",\"uuid\":\"3d735912-8310-49ae-8505-975951f52a87\"},{\"content\":{\"connectorIds\":[\"RConn1\"],\"side\":\"RIGHT\"},\"type\":\"ConnectorPlacement.EquallySpacedRectSide\",\"uuid\":\"85529202-c402-4eb9-9b99-bf632615bd50\"},{\"content\":{\"side\":\"TOP\"},\"type\":\"ConnectorPlacement.EquallySpacedRectSide\",\"uuid\":\"5d103d4e-508a-4997-a1ad-ca112e31789b\"},{\"content\":{\"connectorIds\":[\"Out1\"],\"side\":\"BOTTOM\"},\"type\":\"ConnectorPlacement.EquallySpacedRectSide\",\"uuid\":\"83d15bef-3006-4f95-be48-174a1fa3d22f\"}]},\"type\":\"ConnectorPlacement.EquallySpacedConnector\",\"uuid\":\"22cd4e27-683f-4563-8b2d-583549832478\"}],\"packageUris\":[\"http://schema.mathworks.com/mf0/Connector/R2020b\"],\"version\":\"1.0\"}"
  C : PMIOPort  Side=Right
  P : Outport
  wires:
  Room HVAC/1(S) -> Subsystem/1(S)
  Ts/1 -> Room HVAC/2(Ts)
  Tr/1 -> Room HVAC/1(Tr)
  Subsystem/1(P) -> P/1
  connections:
  Subsystem/RConn1 -- C/RConn1

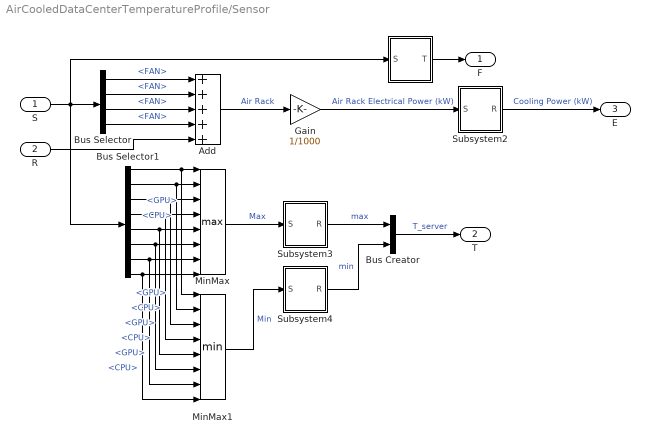
== system AirCooledDataCenterTemperatureProfile/Sensor ==
  S : Inport
  R : Inport  Port=2
  " " : Subsystem
  Add : Sum  Inputs=+++++
  Bus Creator : BusCreator  Inputs=2
  Bus Selector : BusSelector  OutputSignals=D2.FAN,D4.FAN,D3.FAN,D1.FAN
  Bus Selector1 : BusSelector  OutputSignals=D4.GPU,D4.CPU,D3.GPU,D3.CPU,D2.GPU,D2.CPU,D1.GPU,D1.CPU
  Gain : Gain  Gain=1/1000
  MinMax : MinMax  Function=max  Inputs=8
  MinMax1 : MinMax  Inputs=8
  Subsystem2 : Subsystem  mask{sampleTimeSec=1}
      mask prompts: sampleTimeSec "Sample time (s)"
  Subsystem3 : Subsystem  mask{sampleTimeSec=1}
      mask prompts: sampleTimeSec "Sample time (s)"
  Subsystem4 : Subsystem  mask{sampleTimeSec=1}
      mask prompts: sampleTimeSec "Sample time (s)"
  F : Outport
  T : Outport  Port=2
  E : Outport  Port=3
  wires:
  MinMax/1 -> Subsystem3/1(S)  "Max"
  Bus Creator/1 -> T/1  "T_server"
  Gain/1 -> Subsystem2/1(S)  "Air Rack Electrical Power (kW)"
  S/1 -> Bus Selector1/1, Bus Selector/1, " "/1(S)
  MinMax1/1 -> Subsystem4/1(S)  "Min"
  Add/1 -> Gain/1  "Air Rack"
  Bus Selector1/1 -> MinMax1/1, MinMax/1  "<GPU>"
  Bus Selector1/2 -> MinMax1/2, MinMax/2  "<CPU>"
  Bus Selector1/3 -> MinMax1/3, MinMax/3  "<GPU>"
  Bus Selector1/4 -> MinMax1/4, MinMax/4  "<CPU>"
  Bus Selector1/5 -> MinMax1/5, MinMax/5  "<GPU>"
  Bus Selector1/6 -> MinMax1/6, MinMax/6  "<CPU>"
  Bus Selector1/7 -> MinMax1/7, MinMax/7  "<GPU>"
  Bus Selector1/8 -> MinMax1/8, MinMax/8  "<CPU>"
  " "/1(T) -> F/1
  Subsystem2/1(R) -> E/1  "Cooling Power (kW)"
  Subsystem3/1(R) -> Bus Creator/1  "max"
  Subsystem4/1(R) -> Bus Creator/2  "min"
  Bus Selector/1 -> Add/1  "<FAN>"
  Bus Selector/2 -> Add/2  "<FAN>"
  Bus Selector/4 -> Add/4  "<FAN>"
  Bus Selector/3 -> Add/3  "<FAN>"
  R/1 -> Add/5

== system AirCooledDataCenterTemperatureProfile/Subsystem1 ==
  Ambient : fl_lib/Thermal/Thermal Sources/Controlled Temperature Source
  PS-Simulink Converter : nesl_utility/PS-Simulink Converter  PhysicalDomain=network_engine_domain  SubClassName=ps_output  LeftPortType=input  RightPortType=output  PseudoPeriodic=off  Frequencies=[]  VectorFormat=inherit  Unit=inherit  AffineConversion=off
  Thermal Reference : fl_lib/Thermal/Thermal Elements/Thermal Reference
  Thermal Resistance : fl_lib/Thermal/Thermal Elements/Thermal Resistance  resistance=thermalR K/W  T_specify=off  T_priority=None  T=0 K  T_nominal_specify=off  T_nominal_value=1  T_nominal_unit=K  Q_specify=off  Q_priority=None  Q=0 W  Q_nominal_specify=off  Q_nominal_value=1  Q_nominal_unit=W
  Amb : PMIOPort  Side=Left
  T : PMIOPort  Port=2  Side=Left
  Tamb : Outport
  wires:
  PS-Simulink Converter/1 -> Tamb/1  "Ambient"
  connections:
  Thermal Reference/LConn1 -- Ambient/RConn2
  Ambient/LConn1 -- Thermal Resistance/RConn1
  Thermal Resistance/LConn1 -- Amb/RConn1
  T/RConn1 -- PS-Simulink Converter/LConn1 -- Ambient/RConn1

== system AirCooledDataCenterTemperatureProfile/Uvec ==
  Subsystem : Subsystem
  U1 : fl_lib/Physical Signals/Sources/PS Sine Wave  amplitude=0.49  bias=0.5  frequency_spec=foundation.enum.frequencySpec.frequencySI  frequency_SI=1/(6*3600) Hz  frequency_angular=1 rad/s  phase=0 rad
      settings: InternalSimscapePortConfiguration="{\"Bottom\":[],\"Left\":[],\"Right\":[{\"id\":\"O\",\"label\":\"\",\"type\":\"output\"}],\"Top\":[]}"
  U2 : fl_lib/Physical Signals/Sources/PS Sine Wave  amplitude=0.49  bias=0.5  frequency_spec=foundation.enum.frequencySpec.frequencySI  frequency_SI=1/(6*3600) Hz  frequency_angular=1 rad/s  phase=pi/4 rad
      settings: InternalSimscapePortConfiguration="{\"Bottom\":[],\"Left\":[],\"Right\":[{\"id\":\"O\",\"label\":\"\",\"type\":\"output\"}],\"Top\":[]}"
  U3 : fl_lib/Physical Signals/Sources/PS Sine Wave  amplitude=0.49  bias=0.5  frequency_spec=foundation.enum.frequencySpec.frequencySI  frequency_SI=1/(6*3600) Hz  frequency_angular=1 rad/s  phase=pi/2 rad
      settings: InternalSimscapePortConfiguration="{\"Bottom\":[],\"Left\":[],\"Right\":[{\"id\":\"O\",\"label\":\"\",\"type\":\"output\"}],\"Top\":[]}"
  U4 : fl_lib/Physical Signals/Sources/PS Sine Wave  amplitude=0.49  bias=0.5  frequency_spec=foundation.enum.frequencySpec.frequencySI  frequency_SI=1/(6*3600) Hz  frequency_angular=1 rad/s  phase=3*pi/4 rad
      settings: InternalSimscapePortConfiguration="{\"Bottom\":[],\"Left\":[],\"Right\":[{\"id\":\"O\",\"label\":\"\",\"type\":\"output\"}],\"Top\":[]}"
  U : PMIOPort  Side=Right
  connections:
  Subsystem/LConn1 -- U1/RConn1
  Subsystem/LConn2 -- U2/RConn1
  Subsystem/RConn1 -- U/RConn1
  Subsystem/LConn3 -- U3/RConn1
  Subsystem/LConn4 -- U4/RConn1

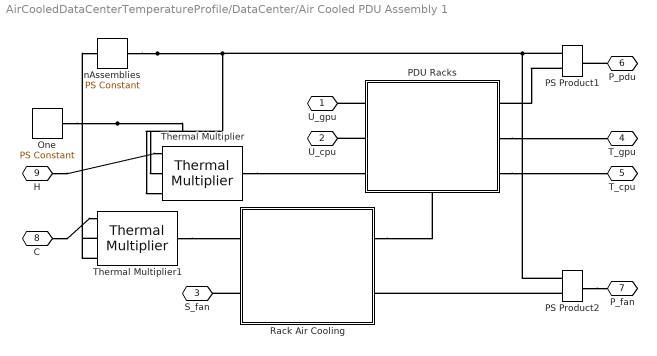
== system AirCooledDataCenterTemperatureProfile/DataCenter/Air Cooled PDU Assembly 1 ==
  One : fl_lib/Physical Signals/Sources/PS Constant  constant=1
  PDU Racks : Subsystem  mask{nTrays=nTrays, nRacks=nRacks, trayMass=trayMass, trayCp=trayCp, trayThermalR=trayThermalR, nGPU=nGPU, gpuTDPperDie=gpuTDPperDie, gpuIdlePower=gpuIdlePower, gpuHBMpower=gpuHBMpower, gpuExponent=gpuExponent, gpuHBMutil=gpuHBMutil, gpuLeakage=gpuLeakage, gpuNominalDieT=gpuNominalDieT, gpuDieThermalC=gpuDieThermalC, gpuHeatSinkR=gpuHeatSinkR, gpuSurfArea=gpuSurfArea, gpuAmbientR=gpuAmbientR, nCPU=nCPU, cpuTDPperSocket=cpuTDPperSocket, cpuIdlePower=cpuIdlePower, cpuExponent=cpuExponent, cpuLeakage=cpuLeakage, cpuNominalDieT=cpuNominalDieT, cpuDieThermalC=cpuDieThermalC, cpuHeatSinkR=cpuHeatSinkR, cpuSurfArea=cpuSurfArea, cpuAmbientR=cpuAmbientR, initialT=initialT, htc=htc}
      mask prompts: nTrays "Number of IT trays per rack (-)"; nRacks "Number of racks (-)"; trayMass "Tray mass (kg)"; trayCp "Tray specific heat capacity (J/kg*K)"; trayThermalR "Tray to external thermal resistance (K/W)"; nGPU "Number of GPU per tray (-)"; gpuTDPperDie "GPU TDP per die (W)"; gpuIdlePower "GPU idle power (W)"; gpuHBMpower "HBM power per GPU (W)"; gpuExponent "GPU power utilization exponent (-)"; gpuHBMutil "HBM utilization as fraction of compute utilization (-)"; gpuLeakage "Leakage increase per K above nominal temperature (W/K)"; gpuNominalDieT "Nominal die temperature at TDP (K)"; gpuDieThermalC "GPU die thermal capacitance (J/K)"; gpuHeatSinkR "GPU die-heat-sink thermal resistance (K/W)"; gpuSurfArea "Surface area per die for ambient heat transfer (m^2)"; gpuAmbientR "GPU die-ambient thermal resistance (K/W)"; nCPU "Number of CPU per tray (-)"; cpuTDPperSocket "CPU TDP per socket (W)"; cpuIdlePower "CPU idle power per socket (W)"; cpuExponent "CPU power utilization exponent (-)"; cpuLeakage "Leakage increase per K above nominal temperature (W/K)"; cpuNominalDieT "Nominal die temperature at TDP (K)"; cpuDieThermalC "CPU die thermal capacitance (J/K)"; cpuHeatSinkR "CPU die-heat-sink thermal resistance (K/W)"; cpuSurfArea "Surface area per die for ambient heat transfer (m^2)"; cpuAmbientR "CPU die-ambient thermal resistance (K/W)"; initialT "Initial temperature (K)"; htc "Heat transfer coefficient to ambient (W/m^2.K)"
      settings: CopyFcn=set_param(gcbh,'LinkStatus','none');  PortSchema="{\"entries\":[{\"content\":{\"sides\":[{\"content\":{\"connectorIds\":[\"LConn1\",\"LConn2\",\"LConn3\"]},\"type\":\"ConnectorPlacement.EquallySpacedRectSide\",\"uuid\":\"1a9a884a-dab1-4495-bf62-c6b2de6c1039\"},{\"content\":{\"connectorIds\":[\"RConn1\",\"RConn2\",\"RConn3\"],\"side\":\"RIGHT\"},\"type\":\"ConnectorPlacement.EquallySpacedRectSide\",\"uuid\":\"05c53434-51c1-4fee-b885-c321dcda8b6b\"},{\"content\":{\"side\":\"TOP\"},\"type\":\"ConnectorPlacement.EquallySpacedRectSide\",\"uuid\":\"c7b5c534-d596-4858-a133-27f005e6c9d4\"},{\"content\":{\"connectorIds\":[\"RConn4\"],\"side\":\"BOTTOM\"},\"type\":\"ConnectorPlacement.EquallySpacedRectSide\",\"uuid\":\"693f3c99-4296-4d86-bfcc-da753d3e576f\"}]},\"type\":\"ConnectorPlacement.EquallySpacedConnector\",\"uuid\":\"ed91c467-c4d0-403f-af16-bac0257594fd\"}],\"packageUris\":[\"http://schema.mathworks.com/mf0/Connector/R2020b\"],\"version\":\"1.0\"}"
      mask Help: web("DocumentationPDURacks.html")
      mask DialogControl Container10 Prompt: PDU Racks
      mask DialogControl getRatingButton Prompt: Get Rating
      mask DialogControl Container9 Prompt: IT Tray
      mask DialogControl Container6 Prompt: GPU
      mask DialogControl Container7 Prompt: CPU
      mask DialogControl Container8 Prompt: Initial Conditions
      mask Display: image('icon_PDURacks.png');
  PS Product1 : fl_lib/Physical Signals/Functions/PS Product
  PS Product2 : fl_lib/Physical Signals/Functions/PS Product
  Rack Air Cooling : Subsystem  mask{nFans=nFans, flowVec=flowVec, prDropVec=prDropVec, fanEffVec=fanEffVec, fluidDen=1.28, fluidCp=1005}
      mask prompts: nFans "Number of fans (-)"; flowVec "Fan flow rate vector (m^3/s)"; prDropVec "Pressure drop vector (Pa)"; fanEffVec "Fan efficiency vector (-)"; fluidDen "Fluid density (kg/m^3)"; fluidCp "Fluid heat capacity (J/(Kg*K))"
      settings: CopyFcn=set_param(gcbh,'LinkStatus','none');
      mask Help: web("DocumentationRackAirCooling.html")
      mask DialogControl Container3 Prompt: Fans
      mask DialogControl Container4 Prompt: Fluid Properties
      mask Display: image('icon_PDUfanCooling.png');
  Thermal Multiplier : datacenter_lib/Thermal Multiplier
      settings: InternalSimscapePortConfiguration="{\"Bottom\":[],\"Left\":[{\"id\":\"A\",\"label\":\"A\",\"type\":\"foundation.thermal.thermal\"}],\"Right\":[{\"id\":\"B\",\"label\":\"B\",\"type\":\"foundation.thermal.thermal\"}],\"Top\":[{\"id\":\"Na\",\"label\":\"Na\",\"type\":\"input\"},{\"id\":\"Nb\",\"label\":\"Nb\",\"type\":\"input\"}]}"
  Thermal Multiplier1 : datacenter_lib/Thermal Multiplier
      settings: InternalSimscapePortConfiguration="{\"Bottom\":[],\"Left\":[{\"id\":\"A\",\"label\":\"A\",\"type\":\"foundation.thermal.thermal\"}],\"Right\":[{\"id\":\"B\",\"label\":\"B\",\"type\":\"foundation.thermal.thermal\"}],\"Top\":[{\"id\":\"Na\",\"label\":\"Na\",\"type\":\"input\"},{\"id\":\"Nb\",\"label\":\"Nb\",\"type\":\"input\"}]}"
  nAssemblies : fl_lib/Physical Signals/Sources/PS Constant  constant=nAssembly
  U_gpu : PMIOPort  Side=Left
  U_cpu : PMIOPort  Port=2  Side=Left
  S_fan : PMIOPort  Port=3  Side=Left
  T_gpu : PMIOPort  Port=4  Side=Right
  T_cpu : PMIOPort  Port=5  Side=Right
  P_pdu : PMIOPort  Port=6  Side=Right
  P_fan : PMIOPort  Port=7  Side=Right
  C : PMIOPort  Port=8  Side=Left
  H : PMIOPort  Port=9  Side=Right
  connections:
  C/RConn1 -- Thermal Multiplier1/LConn1
  H/RConn1 -- Thermal Multiplier/LConn1
  Thermal Multiplier1/RConn1 -- Rack Air Cooling/LConn1
  PS Product2/LConn2 -- Rack Air Cooling/RConn2
  PS Product2/RConn1 -- P_fan/RConn1
  PS Product1/LConn2 -- PDU Racks/RConn1
  P_pdu/RConn1 -- PS Product1/RConn1
  Thermal Multiplier/LConn2 -- Thermal Multiplier1/LConn2 -- One/RConn1
  Thermal Multiplier/LConn3 -- PS Product2/LConn1 -- PS Product1/LConn1 -- Thermal Multiplier1/LConn3 -- nAssemblies/RConn1
  Thermal Multiplier/RConn1 -- PDU Racks/LConn3
  PDU Racks/LConn1 -- U_gpu/RConn1
  Rack Air Cooling/LConn2 -- S_fan/RConn1
  PDU Racks/RConn2 -- T_gpu/RConn1
  PDU Racks/LConn2 -- U_cpu/RConn1
  PDU Racks/RConn3 -- T_cpu/RConn1
  Rack Air Cooling/RConn1 -- PDU Racks/RConn4

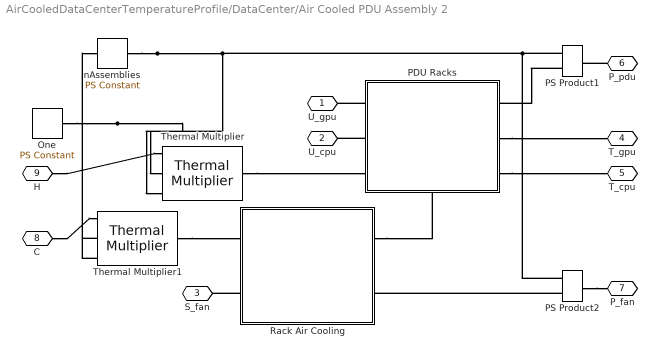
== system AirCooledDataCenterTemperatureProfile/DataCenter/Air Cooled PDU Assembly 2 ==
  One : fl_lib/Physical Signals/Sources/PS Constant  constant=1
  PDU Racks : Subsystem  mask{nTrays=nTrays, nRacks=nRacks, trayMass=trayMass, trayCp=trayCp, trayThermalR=trayThermalR, nGPU=nGPU, gpuTDPperDie=gpuTDPperDie, gpuIdlePower=gpuIdlePower, gpuHBMpower=gpuHBMpower, gpuExponent=gpuExponent, gpuHBMutil=gpuHBMutil, gpuLeakage=gpuLeakage, gpuNominalDieT=gpuNominalDieT, gpuDieThermalC=gpuDieThermalC, gpuHeatSinkR=gpuHeatSinkR, gpuSurfArea=gpuSurfArea, gpuAmbientR=gpuAmbientR, nCPU=nCPU, cpuTDPperSocket=cpuTDPperSocket, cpuIdlePower=cpuIdlePower, cpuExponent=cpuExponent, cpuLeakage=cpuLeakage, cpuNominalDieT=cpuNominalDieT, cpuDieThermalC=cpuDieThermalC, cpuHeatSinkR=cpuHeatSinkR, cpuSurfArea=cpuSurfArea, cpuAmbientR=cpuAmbientR, initialT=initialT, htc=htc}
      mask prompts: nTrays "Number of IT trays per rack (-)"; nRacks "Number of racks (-)"; trayMass "Tray mass (kg)"; trayCp "Tray specific heat capacity (J/kg*K)"; trayThermalR "Tray to external thermal resistance (K/W)"; nGPU "Number of GPU per tray (-)"; gpuTDPperDie "GPU TDP per die (W)"; gpuIdlePower "GPU idle power (W)"; gpuHBMpower "HBM power per GPU (W)"; gpuExponent "GPU power utilization exponent (-)"; gpuHBMutil "HBM utilization as fraction of compute utilization (-)"; gpuLeakage "Leakage increase per K above nominal temperature (W/K)"; gpuNominalDieT "Nominal die temperature at TDP (K)"; gpuDieThermalC "GPU die thermal capacitance (J/K)"; gpuHeatSinkR "GPU die-heat-sink thermal resistance (K/W)"; gpuSurfArea "Surface area per die for ambient heat transfer (m^2)"; gpuAmbientR "GPU die-ambient thermal resistance (K/W)"; nCPU "Number of CPU per tray (-)"; cpuTDPperSocket "CPU TDP per socket (W)"; cpuIdlePower "CPU idle power per socket (W)"; cpuExponent "CPU power utilization exponent (-)"; cpuLeakage "Leakage increase per K above nominal temperature (W/K)"; cpuNominalDieT "Nominal die temperature at TDP (K)"; cpuDieThermalC "CPU die thermal capacitance (J/K)"; cpuHeatSinkR "CPU die-heat-sink thermal resistance (K/W)"; cpuSurfArea "Surface area per die for ambient heat transfer (m^2)"; cpuAmbientR "CPU die-ambient thermal resistance (K/W)"; initialT "Initial temperature (K)"; htc "Heat transfer coefficient to ambient (W/m^2.K)"
      settings: CopyFcn=set_param(gcbh,'LinkStatus','none');  PortSchema="{\"entries\":[{\"content\":{\"sides\":[{\"content\":{\"connectorIds\":[\"LConn1\",\"LConn2\",\"LConn3\"]},\"type\":\"ConnectorPlacement.EquallySpacedRectSide\",\"uuid\":\"1a9a884a-dab1-4495-bf62-c6b2de6c1039\"},{\"content\":{\"connectorIds\":[\"RConn1\",\"RConn2\",\"RConn3\"],\"side\":\"RIGHT\"},\"type\":\"ConnectorPlacement.EquallySpacedRectSide\",\"uuid\":\"05c53434-51c1-4fee-b885-c321dcda8b6b\"},{\"content\":{\"side\":\"TOP\"},\"type\":\"ConnectorPlacement.EquallySpacedRectSide\",\"uuid\":\"c7b5c534-d596-4858-a133-27f005e6c9d4\"},{\"content\":{\"connectorIds\":[\"RConn4\"],\"side\":\"BOTTOM\"},\"type\":\"ConnectorPlacement.EquallySpacedRectSide\",\"uuid\":\"693f3c99-4296-4d86-bfcc-da753d3e576f\"}]},\"type\":\"ConnectorPlacement.EquallySpacedConnector\",\"uuid\":\"ed91c467-c4d0-403f-af16-bac0257594fd\"}],\"packageUris\":[\"http://schema.mathworks.com/mf0/Connector/R2020b\"],\"version\":\"1.0\"}"
      mask Help: web("DocumentationPDURacks.html")
      mask DialogControl Container10 Prompt: PDU Racks
      mask DialogControl getRatingButton Prompt: Get Rating
      mask DialogControl Container9 Prompt: IT Tray
      mask DialogControl Container6 Prompt: GPU
      mask DialogControl Container7 Prompt: CPU
      mask DialogControl Container8 Prompt: Initial Conditions
      mask Display: image('icon_PDURacks.png');
  PS Product1 : fl_lib/Physical Signals/Functions/PS Product
  PS Product2 : fl_lib/Physical Signals/Functions/PS Product
  Rack Air Cooling : Subsystem  mask{nFans=nFans, flowVec=flowVec, prDropVec=prDropVec, fanEffVec=fanEffVec, fluidDen=1.28, fluidCp=1005}
      mask prompts: nFans "Number of fans (-)"; flowVec "Fan flow rate vector (m^3/s)"; prDropVec "Pressure drop vector (Pa)"; fanEffVec "Fan efficiency vector (-)"; fluidDen "Fluid density (kg/m^3)"; fluidCp "Fluid heat capacity (J/(Kg*K))"
      settings: CopyFcn=set_param(gcbh,'LinkStatus','none');
      mask Help: web("DocumentationRackAirCooling.html")
      mask DialogControl Container3 Prompt: Fans
      mask DialogControl Container4 Prompt: Fluid Properties
      mask Display: image('icon_PDUfanCooling.png');
  Thermal Multiplier : datacenter_lib/Thermal Multiplier
      settings: InternalSimscapePortConfiguration="{\"Bottom\":[],\"Left\":[{\"id\":\"A\",\"label\":\"A\",\"type\":\"foundation.thermal.thermal\"}],\"Right\":[{\"id\":\"B\",\"label\":\"B\",\"type\":\"foundation.thermal.thermal\"}],\"Top\":[{\"id\":\"Na\",\"label\":\"Na\",\"type\":\"input\"},{\"id\":\"Nb\",\"label\":\"Nb\",\"type\":\"input\"}]}"
  Thermal Multiplier1 : datacenter_lib/Thermal Multiplier
      settings: InternalSimscapePortConfiguration="{\"Bottom\":[],\"Left\":[{\"id\":\"A\",\"label\":\"A\",\"type\":\"foundation.thermal.thermal\"}],\"Right\":[{\"id\":\"B\",\"label\":\"B\",\"type\":\"foundation.thermal.thermal\"}],\"Top\":[{\"id\":\"Na\",\"label\":\"Na\",\"type\":\"input\"},{\"id\":\"Nb\",\"label\":\"Nb\",\"type\":\"input\"}]}"
  nAssemblies : fl_lib/Physical Signals/Sources/PS Constant  constant=nAssembly
  U_gpu : PMIOPort  Side=Left
  U_cpu : PMIOPort  Port=2  Side=Left
  S_fan : PMIOPort  Port=3  Side=Left
  T_gpu : PMIOPort  Port=4  Side=Right
  T_cpu : PMIOPort  Port=5  Side=Right
  P_pdu : PMIOPort  Port=6  Side=Right
  P_fan : PMIOPort  Port=7  Side=Right
  C : PMIOPort  Port=8  Side=Left
  H : PMIOPort  Port=9  Side=Right
  connections:
  C/RConn1 -- Thermal Multiplier1/LConn1
  H/RConn1 -- Thermal Multiplier/LConn1
  Thermal Multiplier1/RConn1 -- Rack Air Cooling/LConn1
  PS Product2/LConn2 -- Rack Air Cooling/RConn2
  PS Product2/RConn1 -- P_fan/RConn1
  PS Product1/LConn2 -- PDU Racks/RConn1
  P_pdu/RConn1 -- PS Product1/RConn1
  Thermal Multiplier/LConn2 -- Thermal Multiplier1/LConn2 -- One/RConn1
  Thermal Multiplier/LConn3 -- PS Product2/LConn1 -- PS Product1/LConn1 -- Thermal Multiplier1/LConn3 -- nAssemblies/RConn1
  Thermal Multiplier/RConn1 -- PDU Racks/LConn3
  PDU Racks/LConn1 -- U_gpu/RConn1
  Rack Air Cooling/LConn2 -- S_fan/RConn1
  PDU Racks/RConn2 -- T_gpu/RConn1
  PDU Racks/LConn2 -- U_cpu/RConn1
  PDU Racks/RConn3 -- T_cpu/RConn1
  Rack Air Cooling/RConn1 -- PDU Racks/RConn4
